simulink library "Aerodynamics_UL"  (R2019a)
settings: Solver=VariableStepAuto  StartTime=0.0  StopTime=10.0  RelTol=1e-3
undefined symbols (not defined in the file): VEH
libraries: Rail_UL x1
settings Model: Creator=John Jr  LastModifiedBy=jbore

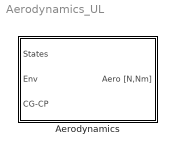
== system Aerodynamics_UL ==
  Aerodynamics : Subsystem  mask{C_d=VEH.C_d, A_ref=VEH.A_ref, C_s=VEH.C_s, A_side=VEH.A_side, z_r=0}
      mask prompts: C_d "Drag Coefficient"; A_ref "Reference area [m^2]"; C_s "Side force coefficient"; A_side "Reference area [m^2]"; z_r "Rail length [m]"
      mask DialogControl DescGroupVar Prompt: Aerodynamics Library
      mask DialogControl DescTextVar Prompt: This block models the aerodynamic forces and moments acting on the vehicle in "body-fixed" coordinates.
      mask DialogControl Control2 Prompt: Drag Force Parameters:
      mask DialogControl Control3 Prompt: Side Force Parameters:
      mask Display:
      | patch([0 1 1 0], [0 0 1 1],[.8 1 1])
      | 
      | port_label('input',1,'\fontname{Cambria Math}States','texmode','on')
      | port_label('input',2,'\fontname{Cambria Math}Env','texmode','on')
      | port_label('input',3,'\fontname{Cambria Math}CP-CG [m]','texmode','on')
      | 
      | port_label('output',1,'\fontname{Cambria Math}Aerodynamics','texmode','on')

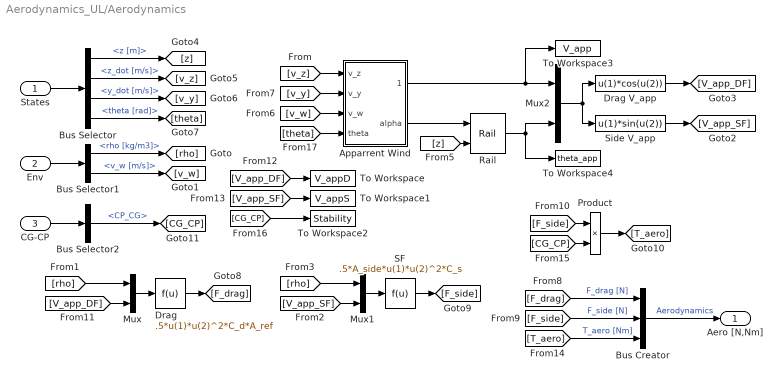
== system Aerodynamics_UL/Aerodynamics ==
  States : Inport
  Env : Inport  Port=2
  CG-CP : Inport  Port=3
  Apparrent Wind : MATLAB Function  TreatAsAtomicUnit=on
  Bus Creator : BusCreator  Inputs=3
  Bus Selector : BusSelector  OutputSignals=Z_g.z [m],Z_g.z_dot [m/s],Y_g.y_dot [m/s],theta.theta [rad]
  Bus Selector1 : BusSelector  OutputSignals=rho [kg/m3],v_w [m/s]
  Bus Selector2 : BusSelector  OutputSignals=CP_CG
  Drag : Fcn  Expr=.5*u(1)*u(2)^2*C_d*A_ref
  Drag V_app : Fcn  Expr=u(1)*cos(u(2))
  Mux : Mux  Inputs=2
  Mux1 : Mux  Inputs=2
  Mux2 : Mux  Inputs=2
  Product : Product
  Rail : Rail_UL/Rail  z_r=ENV.z_r  a_out=0
  SF : Fcn  Expr=.5*A_side*u(1)*u(2)^2*C_s
  Side V_app : Fcn  Expr=u(1)*sin(u(2))
  To Workspace : ToWorkspace  VariableName=V_appD  SampleTime=-1
  To Workspace1 : ToWorkspace  VariableName=V_appS  SampleTime=-1
  To Workspace2 : ToWorkspace  VariableName=Stability  SampleTime=-1
  To Workspace3 : ToWorkspace  VariableName=V_app  SampleTime=-1
  To Workspace4 : ToWorkspace  VariableName=theta_app  SampleTime=-1
  Aero [N,Nm] : Outport
  wires:
  Bus Selector2/1 -> [CG_CP]  "<CP_CG>"
  Drag/1 -> [F_drag]
  [V_app_DF] -> Mux/2
  SF/1 -> [F_side]
  Mux1/1 -> SF/1
  [rho] -> Mux/1
  Mux/1 -> Drag/1
  [rho] -> Mux1/1
  [V_app_SF] -> Mux1/2
  Rail/1 -> To Workspace4/1, Mux2/2
  [v_w] -> Apparrent Wind/3(v_w)
  Side V_app/1 -> [V_app_SF]
  Mux2/1 -> Drag V_app/1, Side V_app/1
  [z] -> Rail/2
  Drag V_app/1 -> [V_app_DF]
  [v_z] -> Apparrent Wind/1(v_z)
  Apparrent Wind/2(alpha) -> Rail/1
  [theta] -> Apparrent Wind/4(theta)
  Apparrent Wind/1(v_app) -> Mux2/1, To Workspace3/1
  [v_y] -> Apparrent Wind/2(v_y)
  [CG_CP] -> To Workspace2/1
  [CG_CP] -> Product/2
  CG-CP/1 -> Bus Selector2/1
  [V_app_SF] -> To Workspace1/1
  [V_app_DF] -> To Workspace/1
  [T_aero] -> Bus Creator/3  "T_aero [Nm]"
  Product/1 -> [T_aero]
  [F_side] -> Product/1
  [F_drag] -> Bus Creator/1  "F_drag [N]"
  [F_side] -> Bus Creator/2  "F_side [N]"
  Bus Creator/1 -> Aero [N,Nm]/1  "Aerodynamics"
  Bus Selector1/2 -> [v_w]  "<v_w [m/s]>"
  Bus Selector1/1 -> [rho]  "<rho [kg/m3]>"
  Env/1 -> Bus Selector1/1
  Bus Selector/4 -> [theta]  "<theta [rad]>"
  Bus Selector/3 -> [v_y]  "<y_dot [m/s]>"
  Bus Selector/2 -> [v_z]  "<z_dot [m/s]>"
  Bus Selector/1 -> [z]  "<z [m]>"
  States/1 -> Bus Selector/1

== matlab function Aerodynamics_UL/Aerodynamics/Apparrent Wind ==
  data: v_z input; v_y input; v_w input; v_app output size=1; alpha output size=1; theta input
function [v_app,alpha] = fcn(v_z,v_y,v_w,theta)

V = [v_y v_z];
V_w = [v_w 0];
V_app = V_w-V;

[theta_V,d_V] = getVangle(V);
if norm(V) == 0
    theta_a = pi/2;
else
    theta_a = acos((-norm(V_w)^2+norm(V)^2+norm(V_app)^2)/(2*norm(V)*norm(V_app)));
end
if V_app(2) > 0
    theta_0 = theta_a-(theta_V*d_V);
else
    theta_0 = theta_a+theta_V*d_V;
end
if V_app(1) >= 0 && V_app(2) <= 0
    alpha = theta_0-theta;
elseif V_app(1) < 0 && V_app(2) <= 0
    alpha = theta_0-theta;
elseif V_app(1) < 0 && V_app(2) > 0
    alpha = -theta_0-theta;
% elseif V_app(1) >= 0 && V_app(2) > 0
else
    alpha = -theta_0-theta;
end
if alpha < -pi
    alpha = 2*pi+alpha;
end
v_app = norm(V_app);
